simulink model "Wind_Turbine"  (R2023a)
settings: Solver=VariableStepAuto  StartTime=0.0  StopTime=10.0  RelTol=1e-3
libraries: spspowerguiLib x1
settings Model: Creator=Dell  LastModifiedBy=Dell

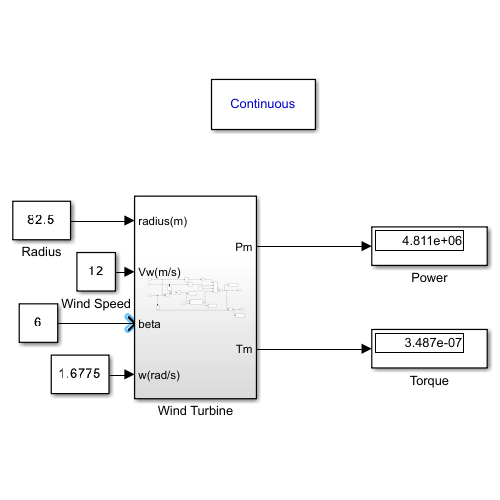
[thumbnail: Simulink's stored preview of the top-level diagram]
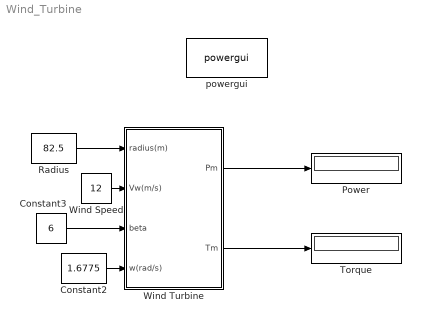
== system Wind_Turbine ==
  Constant2 : Constant  Value=1.6775
  Constant3 : Constant  Value=6
  Power : Display
  Radius : Constant  Value=82.5
  Torque : Display
  Wind Speed : Constant  Value=12
  Wind Turbine : Subsystem
  powergui : spspowerguiLib/powergui  Priority=1  SimulationMode=Continuous  SampleTime=50e-6  frequency=60  Iterations=50  frequencyindice=60  Pbase=100e6  ErrMax=1e-4  UnitsV=kV  UnitsW=MW  buscounter=0  FunctionMessages=off  echomessages=off  EnableUseOfTLC=off  CurrentSourceSwitches=off  DisableSnubberDevices=off  DisableRonSwitches=off  DisableVfSwitches=off  DisplayEquations=off  AutomaticDiscreteSolvers=off  SolverType=Tustin/Backward Euler (TBE)  Interpol=off  ExternalGateDelay=off  methode=off  Ts=100  x0status=blocks  SPID=on  SwTol=0  HookPort=off  NonlinearTolerance=1e-4  nMaxIteration=100  ContinueOnMaxIteration=off  RestoreLinks=warning  ResistiveCurrentMeasurement=off  Frange=[0:2:500]  Ylog=off  Xlog=on  ShowGrid=off  save=off  variable=ZData  structure=0  ZoomFFT=off  StartTime=0.0  cycles=1  DisplayStyle=1  fundamental=60  FreqAxis=off  MaxFrequency=1000  frequencyindicesteady=1  RmsSteady=1  display=off
  wires:
  Constant3/1 -> Wind Turbine/3(beta)
  Wind Speed/1 -> Wind Turbine/2(Vw(m/s))
  Constant2/1 -> Wind Turbine/4(w(rad/s))
  Wind Turbine/2(Tm) -> Torque/1
  Radius/1 -> Wind Turbine/1(radius(m))
  Wind Turbine/1(Pm) -> Power/1

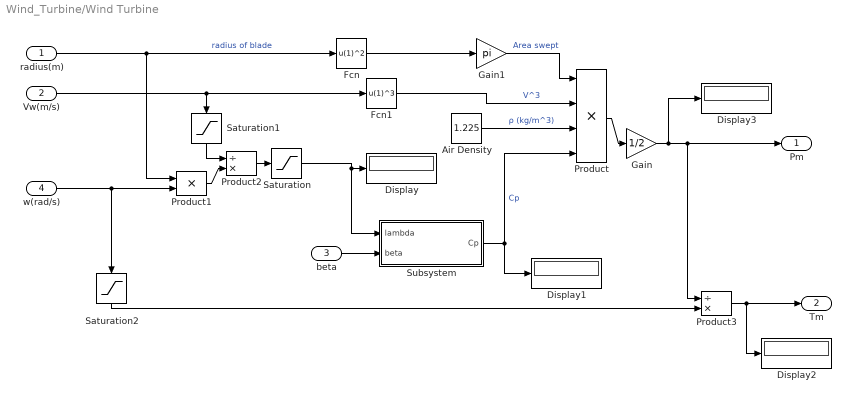
== system Wind_Turbine/Wind Turbine ==
  radius(m) : Inport
  Vw(m/s) : Inport  Port=2
  beta : Inport  Port=3
  w(rad/s) : Inport  Port=4
  Air Density : Constant  Value=1.225
  Display{,1..3} (4 alike) : Display
  Fcn : Fcn  Expr=u(1)^2
  Fcn1 : Fcn  Expr=u(1)^3
  Gain : Gain  Gain=1/2
  Gain1 : Gain  Gain=pi
  Product : Product  Inputs=4
  Product1 : Product
  Product2 : Product  Inputs=/*
  Product3 : Product  Inputs=/*
  Saturation : Saturate  UpperLimit=inf  LowerLimit=1e-6
  Saturation1 : Saturate  UpperLimit=inf  LowerLimit=1e-6
  Saturation2 : Saturate  UpperLimit=inf  LowerLimit=1e-6
  Subsystem : Subsystem
  Pm : Outport
  Tm : Outport  Port=2
  wires:
  Gain/1 -> Display3/1, Pm/1, Product3/1
  Product/1 -> Gain/1
  Fcn1/1 -> Product/2  "V^3"
  Air Density/1 -> Product/3  "ρ (kg/m^3)"
  Subsystem/1(Cp) -> Display1/1, Product/4  "Cp"
  Fcn/1 -> Gain1/1
  Vw(m/s)/1 -> Saturation1/1, Fcn1/1
  beta/1 -> Subsystem/2(beta)
  radius(m)/1 -> Fcn/1, Product1/1  "radius of blade"
  w(rad/s)/1 -> Saturation2/1, Product1/2
  Product1/1 -> Product2/2
  Product2/1 -> Saturation/1
  Saturation/1 -> Display/1, Subsystem/1(lambda)
  Saturation1/1 -> Product2/1
  Saturation2/1 -> Product3/2
  Product3/1 -> Display2/1, Tm/1
  Gain1/1 -> Product/1  "Area swept"

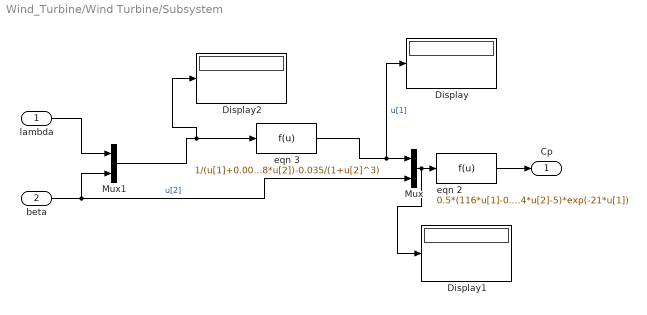
== system Wind_Turbine/Wind Turbine/Subsystem ==
  lambda : Inport
  beta : Inport  Port=2
  Display : Display
  Display1 : Display
  Display2 : Display
  Mux : Mux  Inputs=2
  Mux1 : Mux  Inputs=2
  eqn 2 : Fcn  Expr=0.5*(116*u[1]-0.4*u[2]-5)*exp(-21*u[1])
  eqn 3 : Fcn  Expr=1/(u[1]+0.008*u[2])-0.035/(1+u[2]^3)
  Cp : Outport
  wires:
  eqn 2/1 -> Cp/1
  Mux/1 -> Display1/1, eqn 2/1
  beta/1 -> Mux/2, Mux1/2  "u[2]"
  lambda/1 -> Mux1/1
  eqn 3/1 -> Display/1, Mux/1  "u[1]"
  Mux1/1 -> Display2/1, eqn 3/1
